simulink model "flc_before_case"  (R2018a)
settings: Solver=VariableStepAuto  StartTime=0.0  StopTime=10.0  RelTol=1e-3
libraries: fuzblock x2
settings Model: Creator=Lefteris  LastModifiedBy=Lefteris

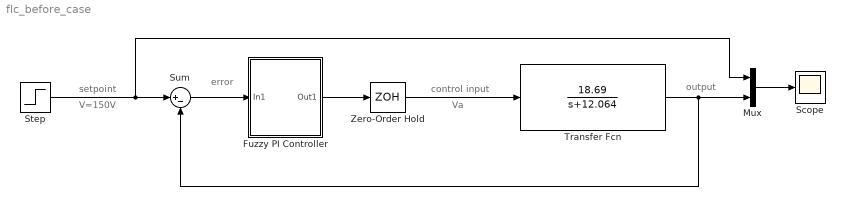
== system flc_before_case ==
  note: output
  note: Va
  note: control input
  note: error
  note: V=150V
  note: setpoint
  Fuzzy PI Controller : Subsystem
  Mux : Mux  Inputs=2
  Scope : Scope
  Step : Step  Time=0  After=150  SampleTime=0.01
  Sum : Sum  Inputs=|+-
  Transfer Fcn : TransferFcn  Numerator=[18.69]  Denominator=[1 12.064]
  Zero-Order Hold : ZeroOrderHold  SampleTime=0.01
  wires:
  Sum/1 -> Fuzzy PI Controller/1(In1)
  Step/1 -> Mux/1, Sum/1
  Fuzzy PI Controller/1(Out1) -> Zero-Order Hold/1
  Zero-Order Hold/1 -> Transfer Fcn/1
  Transfer Fcn/1 -> Sum/2, Mux/2
  Mux/1 -> Scope/1

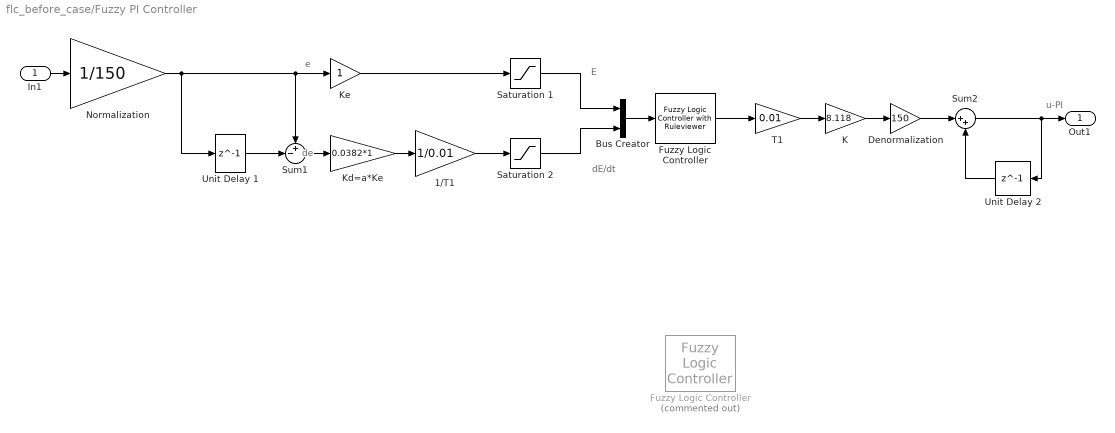
== system flc_before_case/Fuzzy PI Controller ==
  note: u-PI
  note: dE/dt
  note: E
  note: de
  note: e
  In1 : Inport
  1/T1 : Gain  Gain=1/0.01
  Bus Creator : BusCreator  Inputs=2
  "Denormalization " : Gain  Gain=150
  Fuzzy Logic Controller : fuzblock/Fuzzy Logic  Controller  Commented=on  FIS='tipper.fis'  OutputSampleNumber=101  DataType=double  FuzzifiedInputs=off  RuleFiringStrengths=off  RuleOutputs=off  AggregatedOutputs=off  SimulateUsing=Interpreted execution  OutOfRangeInputValueMessage=warning  NoRuleFiredMessage=warning  EmptyOutputFuzzySetMessage=warning
  "Fuzzy Logic Controller " : fuzblock/Fuzzy Logic  Controller  with Ruleviewer  fismatrix=fis  Ts=1
  K : Gain  Gain=8.118
  Kd=a*Ke : Gain  Gain=0.0382*1
  Ke : Gain
  Normalization : Gain  Gain=1/150
  "Saturation 1 " : Saturate  UpperLimit=1  LowerLimit=-1
  "Saturation 2 " : Saturate  UpperLimit=1  LowerLimit=-1
  Sum1 : Sum  Inputs=+-|
  Sum2 : Sum  Inputs=|++
  T1 : Gain  Gain=0.01
  Unit Delay 1 : Delay  DelayLength=1  SampleTime=0.01
  Unit Delay 2 : Delay  DelayLength=1  SampleTime=0.01
  Out1 : Outport
  wires:
  1/T1/1 -> "Saturation 2 "/1
  Kd=a*Ke/1 -> 1/T1/1
  Ke/1 -> "Saturation 1 "/1
  Sum1/1 -> Kd=a*Ke/1
  "Saturation 1 "/1 -> Bus Creator/1
  "Saturation 2 "/1 -> Bus Creator/2
  Unit Delay 2/1 -> Sum2/2
  K/1 -> "Denormalization "/1
  Normalization/1 -> Sum1/1, Ke/1, Unit Delay 1/1
  Unit Delay 1/1 -> Sum1/2
  T1/1 -> K/1
  "Denormalization "/1 -> Sum2/1
  Sum2/1 -> Unit Delay 2/1, Out1/1
  In1/1 -> Normalization/1
  "Fuzzy Logic Controller "/1 -> T1/1
  Bus Creator/1 -> "Fuzzy Logic Controller "/1
